simulink model "lab8_ex3_2018"  (R2018a)
settings: Solver=FixedStepAuto  StartTime=0.0  StopTime=10  FixedStep=0.001  RelTol=1e-3
values from neighbouring files (symbols this model uses):
  A = [-2 0 0 0 0 1 0 0 0 0 4 -3 ... (16 elements, 4x4)]    [lab_8.mat]    (also in laba9_last.m = [5 -7 -5 1)
  B = [0 2 0 5]    [lab_8.mat]    (also in laba9_last.m = [14;10;6;2])
  C = [1 -1 3 3 ... (first row only)    [laba9_last.m]
  K = -Y1*inv(P)    [laba9_last.m]
  L = inv(Q)*Y    [laba9_last.m]
settings Model: Creator=Александр  LastModifiedBy=osini
settings DataIOCC: ReturnWorkspaceOutputs=on
settings DebuggingCC: UnconnectedInputMsg=none  UnconnectedOutputMsg=none  UnconnectedLineMsg=none  SFMachineParentedDataDiag=error
settings SFSimCC: SimUseLocalCustomCode=on
settings RTWCC: RTWUseLocalCustomCode=on

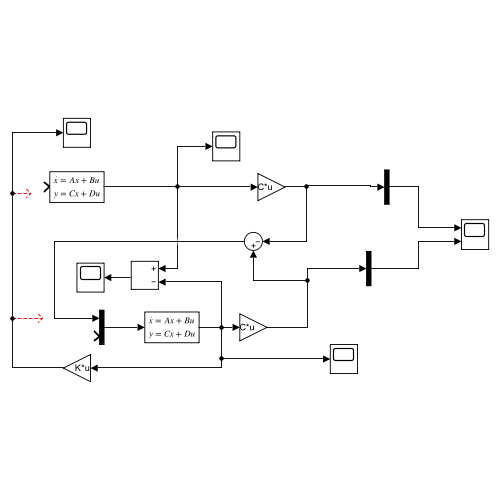
[thumbnail: Simulink's stored preview of the top-level diagram]
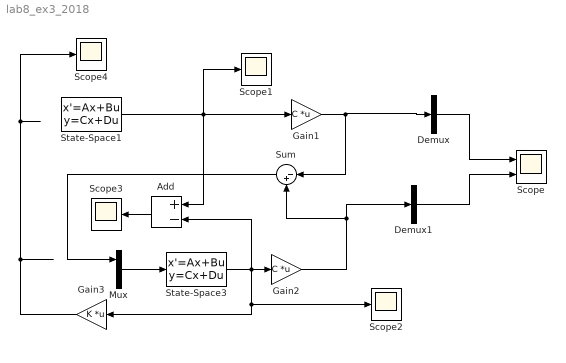
== system lab8_ex3_2018 ==
  Add : Sum  Inputs=+-
  Demux : Demux  Outputs=1
  Demux1 : Demux  Outputs=1
  Gain1 : Gain  Gain=C  Multiplication=Matrix(K*u)
  Gain2 : Gain  Gain=C  Multiplication=Matrix(K*u)
  Gain3 : Gain  Gain=K  Multiplication=Matrix(K*u)
  Mux : Mux  Inputs=2
  Scope : Scope  NumInputPorts=2
  Scope{1..4} (4 alike) : Scope
  State-Space1 : StateSpace  A=A  B=B  C=eye(4,4)  D=[0; 0; 0; 0;]  InitialCondition=[1 1 1 1]'
  State-Space3 : StateSpace  A=A  B=[B L]  C=eye(4,4)  D=[0 0 0; 0 0 0; 0 0 0; 0 0 0]  InitialCondition=[2 0 0 -1]'
  Sum : Sum  Inputs=|-+
  wires:
  Gain1/1 -> Sum/1, Demux/1
  State-Space3/1 -> Gain3/1, Scope2/1, Add/2, Gain2/1
  Gain2/1 -> Demux1/1, Sum/2
  Demux1/1 -> Scope/2
  Mux/1 -> State-Space3/1
  State-Space1/1 -> Add/1, Scope1/1, Gain1/1
  Demux/1 -> Scope/1
  Add/1 -> Scope3/1
  Gain3/1 -> Scope4/1
  Sum/1 -> Mux/1
